simulink model "Subsystem"  (R2020b)
settings: Solver=VariableStepAuto  StartTime=0.0  StopTime=10.0  RelTol=1e-3
settings Model: Creator=Hp  LastModifiedBy=Makrand Raut Dessai
settings DataIOCC: SaveOutput=off  SaveTime=off

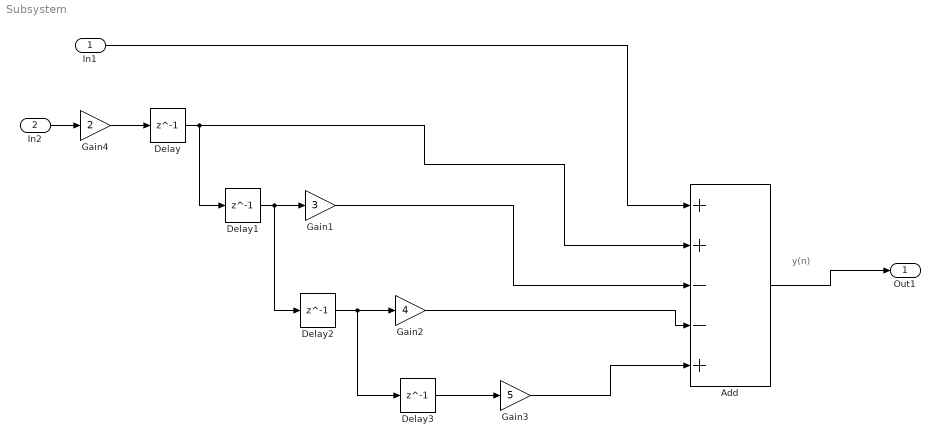
== system Subsystem ==
  note: y(n)
  In1 : Inport  OutDataTypeStr=double  PortDimensions=1  SampleTime=[0,1]
  In2 : Inport  Port=2  OutDataTypeStr=double  PortDimensions=1  SampleTime=[0,1]
  Add : Sum  Inputs=++--+
  Delay{,1..3} (4 alike) : Delay  DelayLength=1
  Gain1 : Gain  Gain=3
  Gain2 : Gain  Gain=4
  Gain3 : Gain  Gain=5
  Gain4 : Gain  Gain=2
  Out1 : Outport  OutDataTypeStr=double  PortDimensions=1  SampleTime=[0,1]
  wires:
  Gain1/1 -> Add/3
  Delay2/1 -> Gain2/1, Delay3/1
  Delay/1 -> Delay1/1, Add/2
  Gain2/1 -> Add/4
  Add/1 -> Out1/1
  Delay1/1 -> Gain1/1, Delay2/1
  Gain4/1 -> Delay/1
  Delay3/1 -> Gain3/1
  Gain3/1 -> Add/5
  In2/1 -> Gain4/1
  In1/1 -> Add/1
